simulink model "set_heave_Eva_Copy"  (R2022b)
settings: Solver=FixedStepAuto  StartTime=0.0  StopTime=7  RelTol=1e-3
values from neighbouring files (symbols this model uses):
  start_position_cm = 10    [command_limits_check.m]    (also in ringdown-circcyl-M10-d0_001-F1-workspace.mat = 0.0117475; setup_CPS_parameters.m = 0)
  T = 0.0002    [ringdown-circcyl-M10-d0_001-F1-workspace.mat]    (also in setup_CPS_parameters.m)
undefined symbols (not defined in the file or in its folder): National_Instruments, PCIe
libraries: sldrtlib x2
settings Model: SimulationMode=external  Creator=eericks1  LastModifiedBy=eericks1
settings DataIOCC: ReturnWorkspaceOutputs=off
settings HardwareCC: ProdBitPerLong=64  ProdHWDeviceType=Intel->x86-64 (Linux 64)
settings RTWCC: Description=Simulink Desktop Real-Time  SystemTargetFile=sldrt.tlc  TemplateMakefile=sldrt.tmf  RTWCompilerOptimization=on
settings CodeAppCC: MaxIdLength=95
settings SimulinkDesktopRealTimeCC: TargetLibSuffix=_sldrt.a  TargetPreCompLibLocation=C:\Program Files\MATLAB\R2022b\toolbox\sldrt\lib\win64

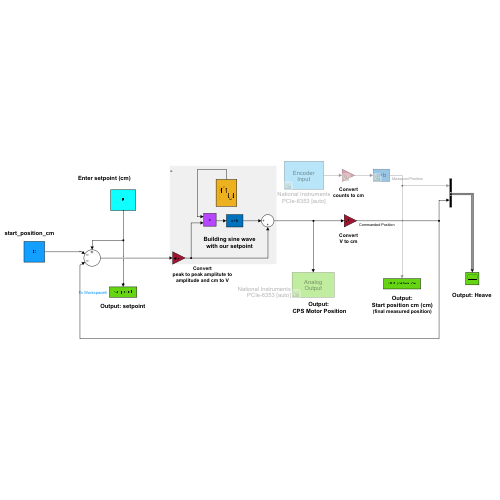
[thumbnail: Simulink's stored preview of the top-level diagram]
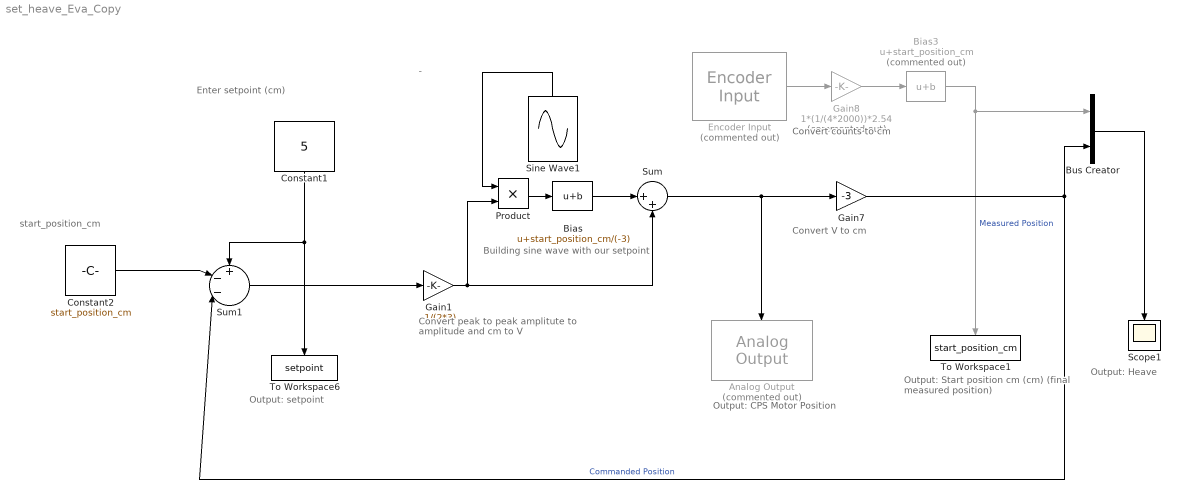
== system set_heave_Eva_Copy ==
  note: Convert
      | counts to cm
  note: Convert
      | V to cm
  note: Output: Heave
  note: Output:
      | CPS Motor Position
  note: Output:
      | Start position cm (cm)
      | (final measured position)
  note: Output: setpoint
  note: Enter setpoint (cm)
  note: start_position_cm
  note: Building sine wave with our setpoint
  note: -
  note: Convert
      | peak to peak amplitute to amplitude and cm to V
  Analog Output : sldrtlib/Analog Output  Commented=on  SampleTime=T  MaxMissedTicks=10  ShowMissedTicks=off  YieldWhenWaiting=off  DrvName=National_Instruments/PCIe-6353  DrvAddress=4294967295  DrvOptions=[0 0 0 2 2 2 2]  Channels=[4]  RangeMode=1  VoltRange=1  InitialValue=[]  FinalValue=[]
      settings: AttributesFormatString=National Instruments\nPCIe-6353 [auto]
  Bias : Bias  Bias=start_position_cm/(-3)  SaturateOnIntegerOverflow=off
  Bias3 : Bias  Commented=on  Bias=start_position_cm  SaturateOnIntegerOverflow=off
  Bus Creator : BusCreator  Inputs=2
  Constant1 : Constant  Value=5
  Constant2 : Constant  Value=start_position_cm  VectorParams1D=off
  Encoder Input : sldrtlib/Encoder Input  Commented=on  SampleTime=T  MaxMissedTicks=10  ShowMissedTicks=off  YieldWhenWaiting=off  DrvName=National_Instruments/PCIe-6353  DrvAddress=4294967295  DrvOptions=[0 0 0 2 2 2 2]  Channels=[1]  QuadMode=3  IndexPulse=1  InputFilter=Inf  DataType=1
      settings: AttributesFormatString=National Instruments\nPCIe-6353 [auto]
  Gain1 : Gain  Gain=-1/(2*3)
  Gain7 : Gain  Gain=-3
  Gain8 : Gain  Commented=on  Gain=1*(1/(4*2000))*2.54
  Product : Product
  Scope1 : Scope
  Sine Wave1 : Sin  Amplitude=-1  Frequency=2*3.14*(1/(2*7))  Phase=pi/2  SampleTime=T
  Sum : Sum  Inputs=|++
  Sum1 : Sum  Inputs=+--|
  To Workspace1 : ToWorkspace  VariableName=start_position_cm  SampleTime=-1
      settings: MaxDataPoints=1  Save2DSignal=2-D array (concatenate along first dimension)
  To Workspace6 : ToWorkspace  VariableName=setpoint  SampleTime=-1
      settings: MaxDataPoints=1  Save2DSignal=2-D array (concatenate along first dimension)
  wires:
  Gain8/1 -> Bias3/1
  Encoder Input/1 -> Gain8/1
  Bias3/1 -> To Workspace1/1, Bus Creator/1  "Measured Position"
  Gain7/1 -> Sum1/3, Bus Creator/2  "Commanded Position"
  Bus Creator/1 -> Scope1/1
  Sum1/1 -> Gain1/1
  Gain1/1 -> Sum/2, Product/2
  Constant1/1 -> To Workspace6/1, Sum1/1
  Sine Wave1/1 -> Product/1
  Product/1 -> Bias/1
  Bias/1 -> Sum/1
  Sum/1 -> Analog Output/1, Gain7/1
  Constant2/1 -> Sum1/2
